simulink model "rozdzielacz_test"  (R2022a)
settings: Solver=ode45  StartTime=0.0  StopTime=180  RelTol=1e-3  EnableMultiTasking=on
undefined symbols (not defined in the file or in its folder): rozdzielacz
libraries: simulink x1
settings Model: Creator=Jarek  LastModifiedBy=bruzd
settings SolverCC: AlgebraicLoopSolver=TrustRegion
settings DataIOCC: LimitDataPoints=on  SaveFormat=Array  SignalLoggingSaveFormat=ModelDataLogs  ReturnWorkspaceOutputs=off
settings OptimizationCC: ExpressionDepthLimit=2147483647  LifeSpan=inf
settings DebuggingCC: UnderspecifiedInitializationDetection=Classic  MergeDetectMultiDrivingBlocksExec=none  SolverPrmCheckMsg=warning  FcnCallInpInsideContextMsg=warning  UnconnectedInputMsg=warning  UnconnectedOutputMsg=warning  UnconnectedLineMsg=warning  StateNameClashWarn=warning  SFUnexpectedBacktrackingDiag=warning  SFNoUnconditionalDefaultTransitionDiag=warning  SFExecutionAtInitializationDiag=none  ArithmeticOperatorsInVariantConditions=warning
settings HardwareCC: ProdBitPerPointer=32  ProdBitPerSizeT=32  ProdBitPerPtrDiffT=32  ProdLargestAtomicFloat=None  ProdIntDivRoundTo=Undefined  ProdEndianess=Unspecified  ProdWordSize=32  ProdHWDeviceType=32-bit Generic
settings ModelReferenceCC: EnableRefExpFcnMdlSchedulingChecks=off  PropagateSignalLabelsOutOfModel=off
settings SFSimCC: SimUseLocalCustomCode=off  CustomCodeUndefinedFunction=UseInterfaceOnly
settings RTWCC: RTWUseLocalCustomCode=off
settings CodeAppCC: StateflowObjectComments=on
settings GRTTargetCC: TargetLangStandard=C89/C90 (ANSI)  CombineOutputUpdateFcns=off  GRTInterface=on
settings ConfigComp: CovMetricSettings=dw  CovSaveCumulativeToWorkspaceVar=on  CovSaveSingleToWorkspaceVar=on  CovExternalEMLEnable=off

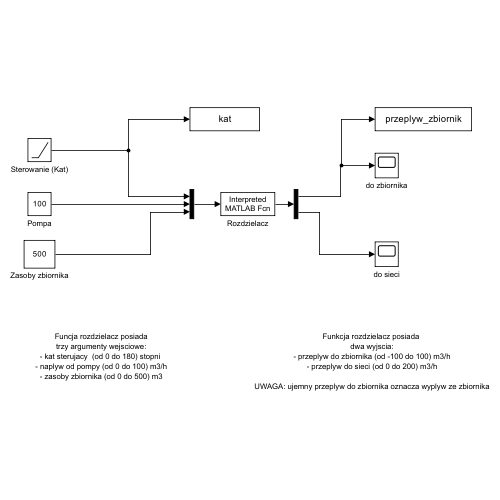
[thumbnail: Simulink's stored preview of the top-level diagram]
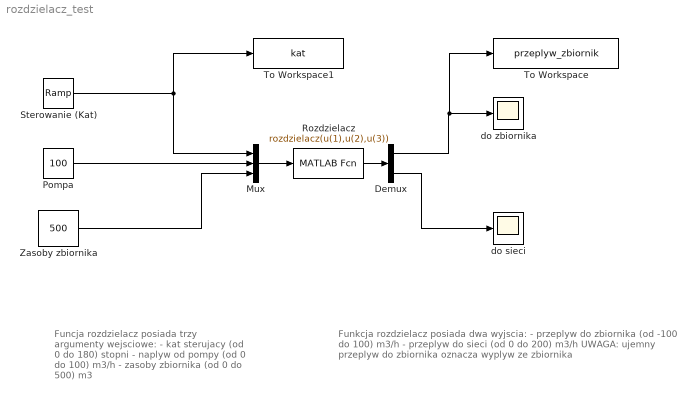
== system rozdzielacz_test ==
  note: Funcja rozdzielacz posiada
      | trzy argumenty wejsciowe:
      | - kat sterujacy  (od 0 do 180) stopni
      | - naplyw od pompy (od 0 do 100) m3/h
      | - zasoby zbiornika (od 0 do 500) m3
  note: Funkcja rozdzielacz posiada
      | dwa wyjscia:
      | - przeplyw do zbiornika (od -100 do 100) m3/h
      | - przeplyw do sieci (od 0 do 200) m3/h
      |
      | UWAGA: ujemny przeplyw do zbiornika oznacza wyplyw ze zbiornika
  Demux : Demux  Outputs=2
  Mux : Mux  Inputs=3
  Pompa : Constant  Value=100
  Rozdzielacz : MATLABFcn  MATLABFcn=rozdzielacz(u(1),u(2),u(3))  OutputDimensions=2
  Sterowanie (Kat) : simulink/Sources/Ramp  slope=1  start=0  InitialOutput=0
  To Workspace : ToWorkspace  VariableName=przeplyw_zbiornik  SaveFormat=Timeseries  SampleTime=-1
  To Workspace1 : ToWorkspace  VariableName=kat  SaveFormat=Timeseries  SampleTime=-1
  Zasoby zbiornika : Constant  Value=500
  do sieci : Scope
  do zbiornika : Scope
  wires:
  Mux/1 -> Rozdzielacz/1
  Pompa/1 -> Mux/2
  Demux/2 -> do sieci/1
  Rozdzielacz/1 -> Demux/1
  Demux/1 -> To Workspace/1, do zbiornika/1
  Zasoby zbiornika/1 -> Mux/3
  Sterowanie (Kat)/1 -> Mux/1, To Workspace1/1
